simulink model "full_sim"  (R2020b)
settings: Solver=FixedStepAuto  StartTime=0.0  StopTime=inf  FixedStep=0.005  RelTol=1e-3
InitFcn:
  | % Load config data automatically
  | load("config.mat");
  | 
  | track = gen_track;
  | map = double(rgb2gray(imread('map.png')));%'iSpaceMapV2.0_50dpi.png')))*100/255;
StartFcn:
  | % The event listener triggers when the signal updates, so we can just monitor one of the signals.
  | blk1 = 'full_sim/GUI_update';
  | 
  | event = 'PostOutputs';
  | listener = @updateApp;
  | 
  | % Create the listener
  | h1 = add_exec_event_listener(blk1, event, listener);
StopFcn:
  | fclose('all') % close any log files that may still be open
model workspace (MAT data in the model file):
  ResetMode = "Reset at each sample time"
  initX = -0.39
  initY = 0.33
  initYaw = 3.14159265359
libraries: simulink x7, simulink_extras x6, dspnetwork x6, pid_lib x2, sldrtlib x1
CloseFcn:
  | fclose('all') % close any log files that may still be open
settings Model: Creator=Duncan  LastModifiedBy=dffleiss
settings DataIOCC: SaveOutput=off  SignalLogging=off  DSMLogging=off  SaveTime=off  ReturnWorkspaceOutputs=off
settings RTWCC: BuildConfiguration=Faster Runs

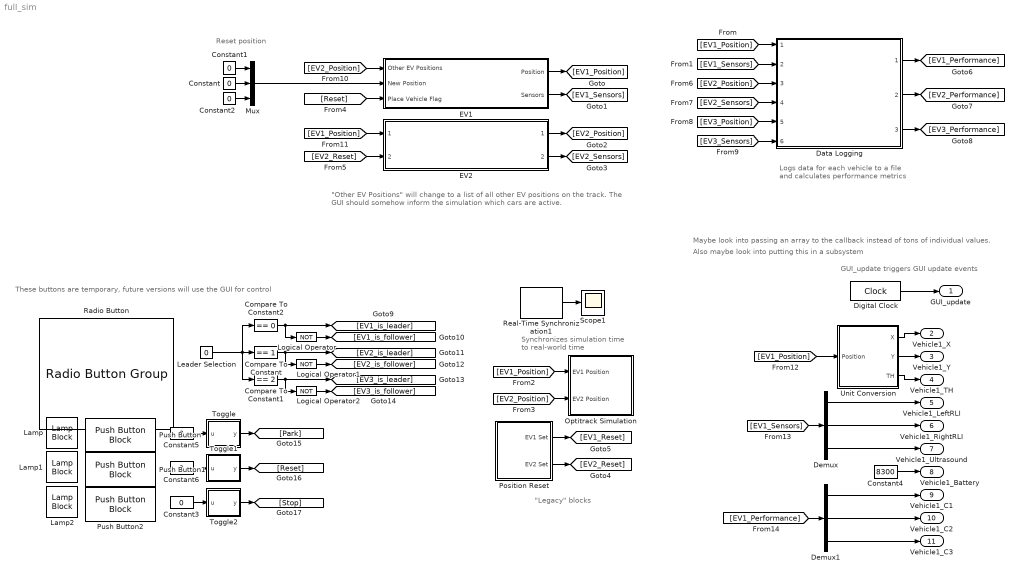
== system full_sim ==
  note: Reset position
  note: These buttons are temporary, future versions will use the GUI for control
  note: "Other EV Positions" will change to a list of all other EV positions on the track.
      | The GUI should somehow inform the simulation which cars are active.
  note: "Legacy" blocks
  note: Synchronizes simulation
      | time to real-world time
  note: Logs data for each vehicle to a file
      | and calculates performance metrics
  note: GUI_update triggers GUI update events
  note: Also maybe look into putting this in a subsystem
  note: Maybe look into passing an array to the callback instead of tons of individual values.
  Compare To Constant : simulink/Logic and Bit Operations/Compare To Constant  relop===  const=1  OutDataTypeStr=boolean
  Compare To Constant1 : simulink/Logic and Bit Operations/Compare To Constant  relop===  const=2  OutDataTypeStr=boolean
  Compare To Constant2 : simulink/Logic and Bit Operations/Compare To Constant  relop===  const=0  OutDataTypeStr=boolean
  Constant{,1..3,5..6} (6 alike) : Constant  Value=0
  Constant4 : Constant  Value=8300
  Data Logging : Subsystem  ReferencedSubsystem=Data_Logging
  Demux : Demux  Outputs=3
  Demux1 : Demux  Outputs=3
  Digital Clock : DigitalClock  SampleTime=0.1
  EV1 : Subsystem
  EV2 : Subsystem  ReferencedSubsystem=Vehicle_Sim  dataTXPort=25004  dataRXPort=25005  cmdPort=25006  initX=0  initY=.33  initYaw=pi  joystickRXPort=25008
  Lamp : LampBlock
  Lamp1 : LampBlock
  Lamp2 : LampBlock
  Leader Selection : Constant  Value=0
  Logical Operator : Logic  Operator=NOT  AllPortsSameDT=off  OutDataTypeStr=boolean
  Logical Operator1 : Logic  Operator=NOT  AllPortsSameDT=off  OutDataTypeStr=boolean
  Logical Operator2 : Logic  Operator=NOT  AllPortsSameDT=off  OutDataTypeStr=boolean
  Mux : Mux  Inputs=3
  Optitrack Simulation : Subsystem
  Position Reset : Subsystem
  Push Button : PushButtonBlock  ButtonText=Park
  Push Button1 : PushButtonBlock  ButtonText=Reset
  Push Button2 : PushButtonBlock  ButtonText=Stop
  Radio Button : RadioButtonGroup  SelectedLabel=EV1 Leader  ButtonGroupName=Group
      settings: Values={{'EV1 Leader', 'EV2 Leader', 'EV3 Leader'}, [0 1 2]}
  Real-Time Synchronization1 : sldrtlib/Real-Time Synchronization  SampleTime=.01  MaxMissedTicks=inf  ShowMissedTicks=on  YieldWhenWaiting=off
  Scope1 : Scope
  Toggle : MATLAB Function  TreatAsAtomicUnit=on
  Toggle1 : MATLAB Function  TreatAsAtomicUnit=on
  Toggle2 : MATLAB Function  TreatAsAtomicUnit=on
  Unit Conversion : Subsystem
  GUI_update : Outport
  Vehicle1_X : Outport  Port=2
  Vehicle1_Y : Outport  Port=3
  Vehicle1_TH : Outport  Port=4
  Vehicle1_LeftRLI : Outport  Port=5
  Vehicle1_RightRLI : Outport  Port=6
  Vehicle1_Ultrasound : Outport  Port=7
  Vehicle1_Battery : Outport  Port=8
  Vehicle1_C1 : Outport  Port=9
  Vehicle1_C2 : Outport  Port=10
  Vehicle1_C3 : Outport  Port=11
  wires:
  [EV2_Position] -> EV1/1(Other EV Positions)
  [EV1_Position] -> EV2/1
  EV2/1 -> [EV2_Position]
  Mux/1 -> EV1/2(New Position)
  EV1/2(Sensors) -> [EV1_Sensors]
  EV1/1(Position) -> [EV1_Position]
  EV2/2 -> [EV2_Sensors]
  Position Reset/2(EV2 Set) -> [EV2_Reset]
  [EV1_Position] -> Optitrack Simulation/1(EV1 Position)
  Position Reset/1(EV1 Set) -> [EV1_Reset]
  [EV2_Position] -> Optitrack Simulation/2(EV2 Position)
  Data Logging/1 -> [EV1_Performance]
  Data Logging/3 -> [EV3_Performance]
  [EV1_Position] -> Data Logging/1
  [EV2_Sensors] -> Data Logging/4
  [EV2_Position] -> Data Logging/3
  [EV3_Position] -> Data Logging/5
  Data Logging/2 -> [EV2_Performance]
  [EV3_Sensors] -> Data Logging/6
  [EV1_Sensors] -> Data Logging/2
  Real-Time Synchronization1/1 -> Scope1/1
  [EV1_Performance] -> Demux1/1
  Demux1/3 -> Vehicle1_C3/1
  Unit Conversion/1(X) -> Vehicle1_X/1
  Demux/2 -> Vehicle1_RightRLI/1
  Unit Conversion/2(Y) -> Vehicle1_Y/1
  Unit Conversion/3(TH) -> Vehicle1_TH/1
  Constant4/1 -> Vehicle1_Battery/1
  Demux1/1 -> Vehicle1_C1/1
  Demux/1 -> Vehicle1_LeftRLI/1
  [EV1_Position] -> Unit Conversion/1(Position)
  Digital Clock/1 -> GUI_update/1
  Demux1/2 -> Vehicle1_C2/1
  [EV1_Sensors] -> Demux/1
  Demux/3 -> Vehicle1_Ultrasound/1
  Constant2/1 -> Mux/3
  Constant/1 -> Mux/2
  Constant1/1 -> Mux/1
  Logical Operator1/1 -> [EV2_is_follower]
  Logical Operator/1 -> [EV1_is_follower]
  Compare To Constant2/1 -> [EV1_is_leader], Logical Operator/1
  Compare To Constant/1 -> [EV2_is_leader], Logical Operator1/1
  Logical Operator2/1 -> [EV3_is_follower]
  Compare To Constant1/1 -> [EV3_is_leader], Logical Operator2/1
  Leader Selection/1 -> Compare To Constant1/1, Compare To Constant2/1, Compare To Constant/1
  Toggle/1(y) -> [Park]
  Constant5/1 -> Toggle/1(u)
  Toggle1/1(y) -> [Reset]
  Constant6/1 -> Toggle1/1(u)
  Toggle2/1(y) -> [Stop]
  Constant3/1 -> Toggle2/1(u)
  [EV2_Reset] -> EV2/2
  [Reset] -> EV1/3(Place Vehicle Flag)

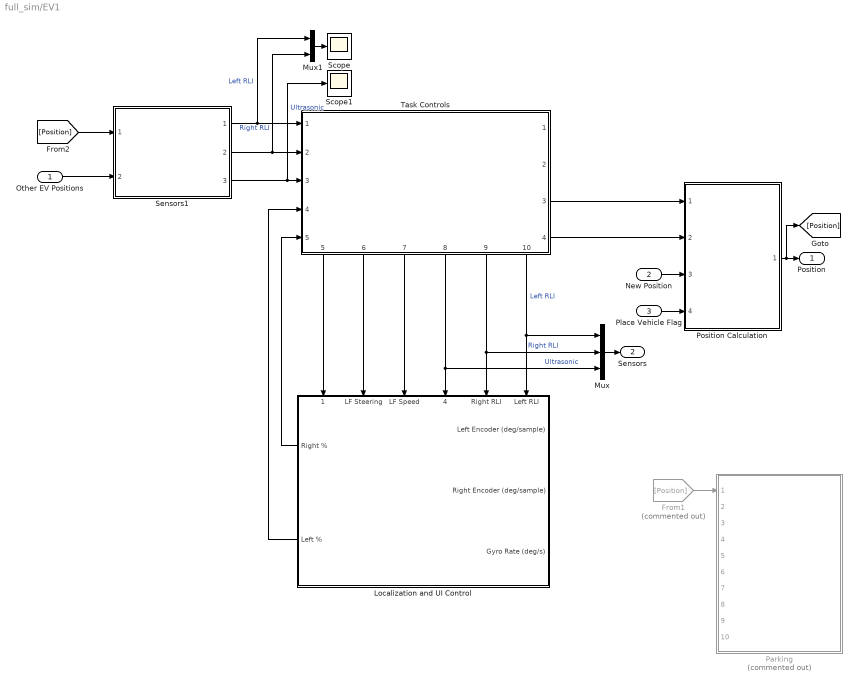
== system full_sim/EV1 ==
  Other EV Positions : Inport
  New Position : Inport  Port=2
  Place Vehicle Flag : Inport  Port=3
  From1 : From  Commented=on  GotoTag=Position
  Localization and UI Control : Subsystem
      settings: PortSchema="{\"entries\":[{\"content\":{\"sides\":[{\"content\":{\"connectorIds\":[\"Out1\",\"Out2\"]},\"type\":\"ConnectorPlacement.EquallySpacedRectSide\",\"uuid\":\"c41f9887-e70f-42cb-a70d-ce479c94e8e6\"},{\"content\":{\"connectorIds\":[\"In7\",\"In8\",\"In9\"],\"side\":\"RIGHT\"},\"type\":\"ConnectorPlacement.EquallySpacedRectSide\",\"uuid\":\"01fea69d-4e07-40c9-8b78-412f64609b36\"},{\"content\":{\"connectorIds\":[\"In1\",\"In2\",\"In3\",\"In4\",\"In5\",\"In6\"],\"side\":\"TOP\"},\"type\":\"ConnectorPlacement.EquallySpacedRectSide\",\"uuid\":\"d2fc7682-afac-46c9-9372-ea085883672c\"}]},\"type\":\"ConnectorPlacement.EquallySpacedConnector\",\"uuid\":\"f49fd9b7-3a1c-45a5-ac31-ef3904fd2313\"}],\"packageUris\":[\"http://schema.mathworks.com/mf0/Connector/19700101\"],\"version\":\"1.0\"}"
  Mux : Mux  Inputs=3
  Mux1 : Mux  Inputs=2
  Parking : Subsystem  Commented=on  ReferencedSubsystem=Parking_ThorneFleissner
  Position Calculation : Subsystem  ReferencedSubsystem=Position_Calculation_ThorneFleissner
  Scope : Scope
  Scope1 : Scope
  Sensors1 : Subsystem  ReferencedSubsystem=Sensors_ThorneFleissner
  Task Controls : Subsystem  ReferencedSubsystem=Task_Controls_ThorneFleissner
      settings: PortSchema="{\"entries\":[{\"content\":{\"sides\":[{\"content\":{\"connectorIds\":[\"In1\",\"In2\",\"In3\",\"In4\",\"In5\"]},\"type\":\"ConnectorPlacement.EquallySpacedRectSide\",\"uuid\":\"3c64813c-625d-49d1-ae67-306451c3c1fa\"},{\"content\":{\"connectorIds\":[\"Out1\",\"Out2\",\"Out3\",\"Out4\"],\"side\":\"RIGHT\"},\"type\":\"ConnectorPlacement.EquallySpacedRectSide\",\"uuid\":\"91793cf5-b7a0-4d71-a2c0-83cdd43afca2\"},{\"content\":{\"connectorIds\":[],\"side\":\"TOP\"},\"type\":\"ConnectorPlacement.EquallySpacedRectSide\",\"uuid\":\"5300aefe-28d7-4142-9759-b53f625cf082\"},{\"content\":{\"connectorIds\":[\"Out5\",\"Out6\",\"Out7\",\"Out8\",\"Out9\",\"Out10\"],\"side\":\"BOTTOM\"},\"type\":\"ConnectorPlacement.EquallySpacedRectSide\",\"uuid\":\"7541b0a2-c079-4b1b-9276-8e4ee5949dfd\"},{\"content\":{\"connectorIds\":[],\"side\":\"HIDDEN\"},\"type\":\"ConnectorPlacement.EquallySpacedRectSide\",\"uuid\":\"d0ef4c96-52b1-4a81-ac1e-c57b650a37a1\"}]},\"type\":\"ConnectorPlacement.EquallySpacedConnector\",\"uuid\":\"d02aae7f-e4d5-4935-81ce-eef5c5855771\"}],\"packageUris\":[\"http://schema.mathworks.com/mf0/Connector/R2020b\"],\"version\":\"1.0\"}"
  Position : Outport
  Sensors : Outport  Port=2
  wires:
  Localization and UI Control/2(Left %) -> Task Controls/4
  Other EV Positions/1 -> Sensors1/2
  Localization and UI Control/1(Right %) -> Task Controls/5
  Task Controls/4 -> Position Calculation/2
  Task Controls/3 -> Position Calculation/1
  Task Controls/7 -> Localization and UI Control/3(LF Speed)
  Task Controls/6 -> Localization and UI Control/2(LF Steering)
  Task Controls/5 -> Localization and UI Control/1(Platoon Speed)
  Task Controls/10 -> Localization and UI Control/6(Left RLI), Mux/1  "Left RLI"
  Task Controls/9 -> Localization and UI Control/5(Right RLI), Mux/2  "Right RLI"
  Task Controls/8 -> Localization and UI Control/4(Ultrasonic (cm)), Mux/3  "Ultrasonic"
  Sensors1/1 -> Mux1/1, Task Controls/1  "Left RLI"
  Sensors1/2 -> Mux1/2, Task Controls/2  "Right RLI"
  Sensors1/3 -> Scope1/1, Task Controls/3  "Ultrasonic"
  Mux/1 -> Sensors/1
  Place Vehicle Flag/1 -> Position Calculation/4
  New Position/1 -> Position Calculation/3
  From1/1 -> Parking/1
  [Position] -> Sensors1/1
  Position Calculation/1 -> [Position], Position/1
  Mux1/1 -> Scope/1

== system full_sim/Optitrack Simulation ==
  EV1 Position : Inport
  EV2 Position : Inport  Port=2
  MATLAB Function : MATLAB Function  TreatAsAtomicUnit=on
  UDP Send : dspnetwork/UDP Send  remoteURL='127.0.0.1'  remotePort=1511  localURL='0.0.0.0'  localPortSource=Automatically determine  localPort=-1  sendBufferSize=8192  sampletime=-1  blockPlatform=[]  separateLengthPort=0
  wires:
  EV1 Position/1 -> MATLAB Function/1(ev1pos)
  EV2 Position/1 -> MATLAB Function/2(ev2pos)
  MATLAB Function/1(packet) -> UDP Send/1

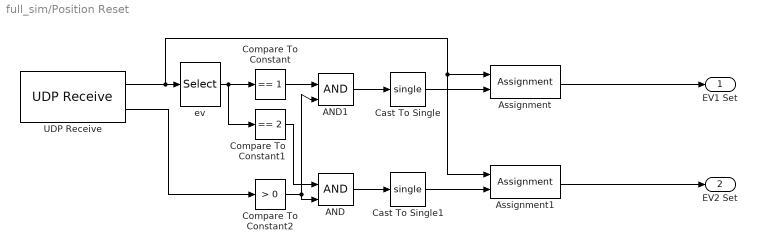
== system full_sim/Position Reset ==
  AND : Logic  IconShape=distinctive  AllPortsSameDT=off  OutDataTypeStr=boolean
  AND1 : Logic  IconShape=distinctive  AllPortsSameDT=off  OutDataTypeStr=boolean
  Assignment : Assignment  DiagnosticForDimensions=Warning  IndexOptions=Index vector (dialog)  Indices=1  OutputSizes=1
  Assignment1 : Assignment  DiagnosticForDimensions=Warning  IndexOptions=Index vector (dialog)  Indices=1  OutputSizes=1
  Cast To Single : DataTypeConversion  OutDataTypeStr=single
  Cast To Single1 : DataTypeConversion  OutDataTypeStr=single
  Compare To Constant : simulink/Logic and Bit Operations/Compare To Constant  relop===  const=1  OutDataTypeStr=boolean
  Compare To Constant1 : simulink/Logic and Bit Operations/Compare To Constant  relop===  const=2  OutDataTypeStr=boolean
  Compare To Constant2 : simulink/Logic and Bit Operations/Compare To Constant  relop=>  const=0  OutDataTypeStr=boolean
  UDP Receive : dspnetwork/UDP Receive  localURL='0.0.0.0'  localPort=24999  remoteURL='0.0.0.0'  remotePort=-1  recvBufferSize=512  dims=4  signalDatatype=single  isComplex=off  isVarSize=off  showBlockingTime=off  blockingTime=0  sampletime=0.01  blockPlatform=[]
  ev : Selector  InputPortWidth=4  IndexOptions=Index vector (dialog)  Indices=[1]  OutputSizes=1
  EV1 Set : Outport
  EV2 Set : Outport  Port=2
  wires:
  Compare To Constant2/1 -> AND1/2, AND/2
  UDP Receive/2 -> Compare To Constant2/1
  ev/1 -> Compare To Constant1/1, Compare To Constant/1
  Assignment/1 -> EV1 Set/1
  Compare To Constant/1 -> AND1/1
  Assignment1/1 -> EV2 Set/1
  UDP Receive/1 -> Assignment/1, Assignment1/1, ev/1
  AND/1 -> Cast To Single1/1
  Compare To Constant1/1 -> AND/1
  Cast To Single/1 -> Assignment/2
  AND1/1 -> Cast To Single/1
  Cast To Single1/1 -> Assignment1/2

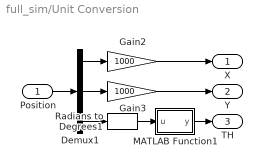
== system full_sim/Unit Conversion ==
  Position : Inport
  Demux1 : Demux  Outputs=3
  Gain2 : Gain  Gain=1000
  Gain3 : Gain  Gain=1000
  MATLAB Function1 : MATLAB Function  TreatAsAtomicUnit=on
  Radians to Degrees1 : simulink_extras/Transformations/Radians to Degrees
  X : Outport
  Y : Outport  Port=2
  TH : Outport  Port=3
  wires:
  Radians to Degrees1/1 -> MATLAB Function1/1(u)
  Gain3/1 -> Y/1
  Demux1/3 -> Radians to Degrees1/1
  Demux1/2 -> Gain3/1
  Gain2/1 -> X/1
  MATLAB Function1/1(y) -> TH/1
  Demux1/1 -> Gain2/1
  Position/1 -> Demux1/1

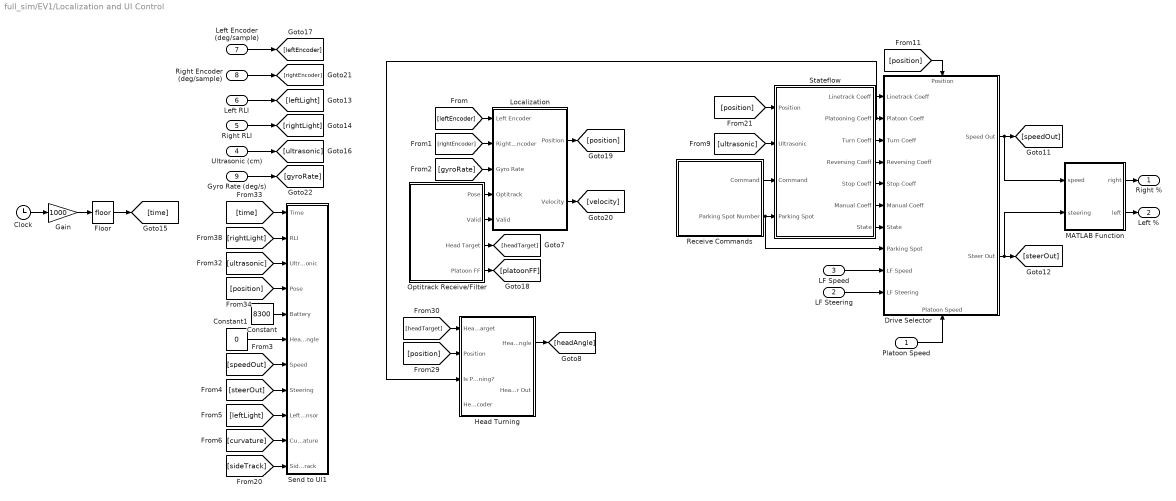
== system full_sim/EV1/Localization and UI Control ==
  Platoon Speed : Inport
  LF Steering : Inport  Port=2
  LF Speed : Inport  Port=3
  Ultrasonic (cm) : Inport  Port=4
  Right RLI : Inport  Port=5
  Left RLI : Inport  Port=6
  Left Encoder (deg/sample) : Inport  Port=7
  Right Encoder (deg/sample) : Inport  Port=8
  Gyro Rate (deg/s) : Inport  Port=9
  Clock : Clock
  Constant : Constant  Value=8300
  Constant1 : Constant  Value=0
  Drive Selector : Subsystem
      settings: PortSchema="{\"entries\":[{\"content\":{\"sides\":[{\"content\":{\"connectorIds\":[\"In1\",\"In2\",\"In3\",\"In4\",\"In5\",\"In6\",\"In7\",\"In8\",\"In9\",\"In10\"]},\"type\":\"ConnectorPlacement.EquallySpacedRectSide\",\"uuid\":\"ae307232-287c-4602-bc59-e7aee20cf720\"},{\"content\":{\"connectorIds\":[\"Out1\",\"Out2\"],\"side\":\"RIGHT\"},\"type\":\"ConnectorPlacement.EquallySpacedRectSide\",\"uuid\":\"2cae2544-d808-4029-9530-a1f56251b9cd\"},{\"content\":{\"connectorIds\":[\"In11\"],\"side\":\"TOP\"},\"type\":\"ConnectorPlacement.EquallySpacedRectSide\",\"uuid\":\"bbc0be7b-0147-487e-824e-99eef1e06dcc\"},{\"content\":{\"connectorIds\":[\"In12\"],\"side\":\"BOTTOM\"},\"type\":\"ConnectorPlacement.EquallySpacedRectSide\",\"uuid\":\"b1fbed80-afe2-48db-af11-c85938407aae\"}]},\"type\":\"ConnectorPlacement.EquallySpacedConnector\",\"uuid\":\"38f7d747-6147-4f1b-8575-02c2e0fe0660\"}],\"packageUris\":[\"http://schema.mathworks.com/mf0/Connector/19700101\"],\"version\":\"1.0\"}"
  Floor : Rounding
  Gain : Gain  Gain=1000
  Head Turning : Subsystem
  Localization : Subsystem
  MATLAB Function : MATLAB Function  TreatAsAtomicUnit=on
  Optitrack Receive/Filter : Subsystem
  Receive Commands : Subsystem
  Send to UI1 : Subsystem
  Stateflow : Subsystem
  Right % : Outport
  Left % : Outport  Port=2
  wires:
  Constant/1 -> Send to UI1/5(Battery)
  [position] -> Head Turning/2(Position)
  Left RLI/1 -> [leftLight]
  Localization/2(Velocity) -> [velocity]
  Stateflow/6(Manual Coeff) -> Drive Selector/6(Manual Coeff)
  [leftEncoder] -> Localization/1(Left Encoder)
  MATLAB Function/1(right) -> Right %/1
  Head Turning/1(Head Angle) -> [headAngle]
  Optitrack Receive/Filter/4(Platoon FF) -> [platoonFF]
  [gyroRate] -> Localization/3(Gyro Rate)
  Floor/1 -> [time]
  Drive Selector/2(Steer Out) -> [steerOut], MATLAB Function/2(steering)
  Optitrack Receive/Filter/2(Valid) -> Localization/5(Valid)
  Clock/1 -> Gain/1
  Right Encoder (deg/sample)/1 -> [rightEncoder]
  Optitrack Receive/Filter/3(Head Target) -> [headTarget]
  Left Encoder (deg/sample)/1 -> [leftEncoder]
  Gain/1 -> Floor/1
  Receive Commands/1(Command) -> Stateflow/3(Command)
  [ultrasonic] -> Send to UI1/3(Ultrasonic)
  [curvature] -> Send to UI1/10(Curvature)
  Stateflow/4(Reversing Coeff) -> Drive Selector/4(Reversing Coeff)
  Gyro Rate (deg/s)/1 -> [gyroRate]
  [leftLight] -> Send to UI1/9(Left Sensor)
  [sideTrack] -> Send to UI1/11(Side Track)
  Drive Selector/1(Speed Out) -> [speedOut], MATLAB Function/1(speed)
  Right RLI/1 -> [rightLight]
  Ultrasonic (cm)/1 -> [ultrasonic]
  MATLAB Function/2(left) -> Left %/1
  [speedOut] -> Send to UI1/7(Speed)
  [steerOut] -> Send to UI1/8(Steering)
  Stateflow/7(State) -> Drive Selector/7(State)
  Stateflow/5(Stop Coeff) -> Drive Selector/5(Stop Coeff)
  Localization/1(Position) -> [position]
  Optitrack Receive/Filter/1(Pose) -> Localization/4(Optitrack)
  [position] -> Send to UI1/4(Pose)
  Stateflow/3(Turn Coeff) -> Drive Selector/3(Turn Coeff)
  [rightLight] -> Send to UI1/2(RLI)
  Stateflow/2(Platooning Coeff) -> Head Turning/3(Is Platooning?), Drive Selector/2(Platoon Coeff)
  [ultrasonic] -> Stateflow/2(Ultrasonic)
  [headTarget] -> Head Turning/1(Head Target)
  [position] -> Stateflow/1(Position)
  Stateflow/1(Linetrack Coeff) -> Drive Selector/1(Linetrack Coeff)
  Receive Commands/2(Parking Spot Number) -> Drive Selector/8(Parking Spot), Stateflow/4(Parking Spot)
  [position] -> Drive Selector/11(Position)
  [rightEncoder] -> Localization/2(Right Encoder)
  [time] -> Send to UI1/1(Time)
  Constant1/1 -> Send to UI1/6(Head Angle)
  LF Speed/1 -> Drive Selector/9(LF Speed)
  LF Steering/1 -> Drive Selector/10(LF Steering)
  Platoon Speed/1 -> Drive Selector/12(Platoon Speed)

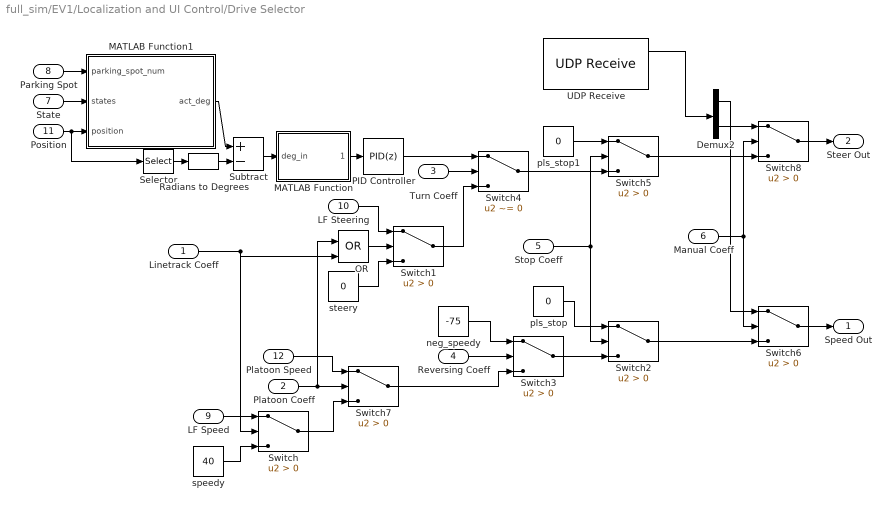
== system full_sim/EV1/Localization and UI Control/Drive Selector ==
  Linetrack Coeff : Inport
  Platoon Coeff : Inport  Port=2
  Turn Coeff : Inport  Port=3
  Reversing Coeff : Inport  Port=4
  Stop Coeff : Inport  Port=5
  Manual Coeff : Inport  Port=6
  State : Inport  Port=7
  Parking Spot : Inport  Port=8
  LF Speed : Inport  Port=9
  LF Steering : Inport  Port=10
  Position : Inport  Port=11
  Platoon Speed : Inport  Port=12
  Demux2 : Demux  Outputs=2
  MATLAB Function : MATLAB Function  TreatAsAtomicUnit=on
  MATLAB Function1 : MATLAB Function  TreatAsAtomicUnit=on
  OR : Logic  Operator=OR  IconShape=distinctive  AllPortsSameDT=off  OutDataTypeStr=boolean
  PID Controller : pid_lib/PID Controller  Controller=PID  Form=Parallel  TimeDomain=Discrete-time  UseExternalTs=off  SampleTime=-1  IntegratorMethod=Forward Euler  FilterMethod=Forward Euler  ControllerParametersSource=internal  P=1  I=0  D=0  UseFilter=off  N=100  TunerSelectOption=Transfer Function Based (PID Tuner App)  InitialConditionSource=internal  InitialConditionForIntegrator=0  InitialConditionForFilter=0  DifferentiatorICPrevScaledInput=0  ExternalReset=none  TrackingMode=off  Kt=1  LimitOutput=off  SatLimitsSource=internal  UpperSaturationLimit=inf  LowerSaturationLimit=-inf  LinearizeAsGain=on  AntiWindupMode=none  Kb=1  POutMin=[]  POutMax=[]  IOutMin=[]  IOutMax=[]  DOutMin=[]  DOutMax=[]  NOutMin=[]  NOutMax=[]  SumOutMin=[]  SumOutMax=[]  SaturationOutMin=[]  SaturationOutMax=[]  PParamMin=[]  PParamMax=[]  IParamMin=[]  IParamMax=[]  DParamMin=[]  DParamMax=[]  NParamMin=[]  NParamMax=[]  KbParamMin=[]  KbParamMax=[]  KtParamMin=[]  KtParamMax=[]  KbOutMin=[]  KbOutMax=[]  KtOutMin=[]  KtOutMax=[]  IntegratorOutMin=[]  IntegratorOutMax=[]  FilterOutMin=[]  FilterOutMax=[]  SumI1OutMin=[]  SumI1OutMax=[]  SumI2OutMin=[]  SumI2OutMax=[]  SumI3OutMin=[]  SumI3OutMax=[]  SumI4OutMin=[]  SumI4OutMax=[]  SumDOutMin=[]  SumDOutMax=[]  DifferentiatorOutMin=[]  DifferentiatorOutMax=[]  FilterDiffOutCoefMin=[]  FilterDiffOutCoefMax=[]  ReciprocalOutMin=[]  ReciprocalOutMax=[]  SumDenOutMin=[]  SumDenOutMax=[]  SumNumOutMin=[]  SumNumOutMax=[]  DivideOutMin=[]  DivideOutMax=[]  UdiffTsProdOutMin=[]  UdiffTsProdOutMax=[]  NTsProdOutMin=[]  NTsProdOutMax=[]  UintegralTsProdOutMin=[]  UintegralTsProdOutMax=[]  UngainTsProdOutMin=[]  UngainTsProdOutMax=[]  IntegratorContinuousStateAttributes=''  IntegratorStateMustResolveToSignalObject=off  IntegratorRTWStateStorageClass=Auto  FilterContinuousStateAttributes=''  FilterStateMustResolveToSignalObject=off  FilterRTWStateStorageClass=Auto  ParallelPVariant=InternalParameters  IdealPVariant=Disabled  IVariant=InternalParameters  DVariant=InternalParameters  IntegratorVariant=Discrete  SatVariant=Disabled  AWVariant=Passthrough  PCopyVariant=Disabled  TRVariant=Disabled  FdbkBlocksVariant=Forward  IdealPFdbkVariant=Disabled  SatFdbkVariant=Disabled  DerivativeFilterVariant=Differentiator  NVariant=Passthrough  NCopyVariant=Disabled_SignalSpec  FilterICVariant=InternalICsDifferentiator  IntegratorICVariant=InternalICs  ExternalResetVariant=Disabled  TRSumVariant=Passthrough  SumFdbkVariant=Disabled  SumVariant=Sum_PID  TsampFilterVariant=InternalTs  TsampNgainVariant=Passthrough  TsampIntegralVariant=Passthrough  ExternalSaturationOutDataTypeStr=Inherit: Same as second input
  Radians to Degrees : simulink_extras/Transformations/Radians to Degrees
  Selector : Selector  InputPortWidth=3  IndexOptions=Index vector (dialog)  Indices=[3]  OutputSizes=1
  Subtract : Sum  Inputs=+-
  Switch{,1..3,5..8} (8 alike) : Switch  Criteria=u2 > Threshold
  Switch4 : Switch  Criteria=u2 ~= 0
  UDP Receive : dspnetwork/UDP Receive  localURL='0.0.0.0'  localPort=joystickRXPort  remoteURL='0.0.0.0'  remotePort=-1  recvBufferSize=384  dims=2  signalDatatype=single  isComplex=off  isVarSize=off  showBlockingTime=off  blockingTime=0  sampletime=0.01  blockPlatform=[]
  neg_speedy : Constant  Value=-75
  pls_stop : Constant  Value=0
  pls_stop1 : Constant  Value=0
  speedy : Constant  Value=40
  steery : Constant  Value=0
  Speed Out : Outport
  Steer Out : Outport  Port=2
  wires:
  Demux2/1 -> Switch6/1
  Demux2/2 -> Switch8/1
  Switch6/1 -> Speed Out/1
  Switch8/1 -> Steer Out/1
  Manual Coeff/1 -> Switch6/2, Switch8/2
  Switch2/1 -> Switch6/3
  Switch5/1 -> Switch8/3
  UDP Receive/1 -> Demux2/1
  LF Speed/1 -> Switch/1
  LF Steering/1 -> Switch1/1
  steery/1 -> Switch1/3
  speedy/1 -> Switch/3
  Switch1/1 -> Switch4/3
  Switch3/1 -> Switch2/3
  Stop Coeff/1 -> Switch2/2, Switch5/2
  pls_stop/1 -> Switch2/1
  Turn Coeff/1 -> Switch4/2
  PID Controller/1 -> Switch4/1
  Subtract/1 -> MATLAB Function/1(deg_in)
  MATLAB Function/1(deg_out) -> PID Controller/1
  Radians to Degrees/1 -> Subtract/2
  Parking Spot/1 -> MATLAB Function1/1(parking_spot_num)
  Reversing Coeff/1 -> Switch3/2
  State/1 -> MATLAB Function1/2(states)
  Position/1 -> Selector/1, MATLAB Function1/3(position)
  Switch4/1 -> Switch5/3
  neg_speedy/1 -> Switch3/1
  MATLAB Function1/1(act_deg) -> Subtract/1
  OR/1 -> Switch1/2
  Platoon Coeff/1 -> OR/1, Switch7/2
  Linetrack Coeff/1 -> Switch/2, OR/2
  Switch7/1 -> Switch3/3
  Switch/1 -> Switch7/3
  Selector/1 -> Radians to Degrees/1
  pls_stop1/1 -> Switch5/1
  Platoon Speed/1 -> Switch7/1

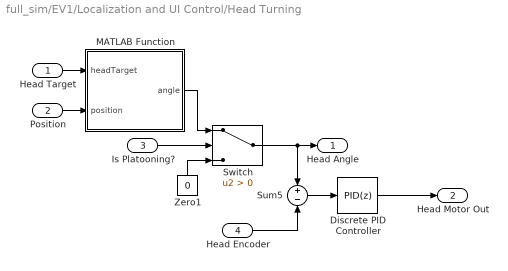
== system full_sim/EV1/Localization and UI Control/Head Turning ==
  Head Target : Inport
  Position : Inport  Port=2
  Is Platooning? : Inport  Port=3
  Head Encoder : Inport  Port=4
  Discrete PID Controller : pid_lib/PID Controller  Controller=PID  Form=Parallel  TimeDomain=Discrete-time  UseExternalTs=off  SampleTime=-1  IntegratorMethod=Forward Euler  FilterMethod=Forward Euler  ControllerParametersSource=internal  P=1  I=1  D=0  UseFilter=off  N=100  TunerSelectOption=Transfer Function Based (PID Tuner App)  InitialConditionSource=internal  InitialConditionForIntegrator=0  InitialConditionForFilter=0  DifferentiatorICPrevScaledInput=0  ExternalReset=none  TrackingMode=off  Kt=1  LimitOutput=off  SatLimitsSource=internal  UpperSaturationLimit=inf  LowerSaturationLimit=-inf  LinearizeAsGain=off  AntiWindupMode=none  Kb=1  POutMin=[]  POutMax=[]  IOutMin=[]  IOutMax=[]  DOutMin=[]  DOutMax=[]  NOutMin=[]  NOutMax=[]  SumOutMin=[]  SumOutMax=[]  SaturationOutMin=[]  SaturationOutMax=[]  PParamMin=[]  PParamMax=[]  IParamMin=[]  IParamMax=[]  DParamMin=[]  DParamMax=[]  NParamMin=[]  NParamMax=[]  KbParamMin=[]  KbParamMax=[]  KtParamMin=[]  KtParamMax=[]  KbOutMin=[]  KbOutMax=[]  KtOutMin=[]  KtOutMax=[]  IntegratorOutMin=[]  IntegratorOutMax=[]  FilterOutMin=[]  FilterOutMax=[]  SumI1OutMin=[]  SumI1OutMax=[]  SumI2OutMin=[]  SumI2OutMax=[]  SumI3OutMin=[]  SumI3OutMax=[]  SumI4OutMin=[]  SumI4OutMax=[]  SumDOutMin=[]  SumDOutMax=[]  DifferentiatorOutMin=[]  DifferentiatorOutMax=[]  FilterDiffOutCoefMin=[]  FilterDiffOutCoefMax=[]  ReciprocalOutMin=[]  ReciprocalOutMax=[]  SumDenOutMin=[]  SumDenOutMax=[]  SumNumOutMin=[]  SumNumOutMax=[]  DivideOutMin=[]  DivideOutMax=[]  UdiffTsProdOutMin=[]  UdiffTsProdOutMax=[]  NTsProdOutMin=[]  NTsProdOutMax=[]  UintegralTsProdOutMin=[]  UintegralTsProdOutMax=[]  UngainTsProdOutMin=[]  UngainTsProdOutMax=[]  IntegratorContinuousStateAttributes=''  IntegratorStateMustResolveToSignalObject=off  IntegratorRTWStateStorageClass=Auto  FilterContinuousStateAttributes=''  FilterStateMustResolveToSignalObject=off  FilterRTWStateStorageClass=Auto  ParallelPVariant=InternalParameters  IdealPVariant=Disabled  IVariant=InternalParameters  DVariant=InternalParameters  IntegratorVariant=Discrete  SatVariant=Disabled  AWVariant=Passthrough  PCopyVariant=Disabled  TRVariant=Disabled  FdbkBlocksVariant=Forward  IdealPFdbkVariant=Disabled  SatFdbkVariant=Disabled  DerivativeFilterVariant=Differentiator  NVariant=Passthrough  NCopyVariant=Disabled_SignalSpec  FilterICVariant=InternalICsDifferentiator  IntegratorICVariant=InternalICs  ExternalResetVariant=Disabled  TRSumVariant=Passthrough  SumFdbkVariant=Disabled  SumVariant=Sum_PID  TsampFilterVariant=InternalTs  TsampNgainVariant=Passthrough  TsampIntegralVariant=Passthrough  ExternalSaturationOutDataTypeStr=Inherit: Same as second input
  MATLAB Function : MATLAB Function  TreatAsAtomicUnit=on
  Sum5 : Sum  Inputs=+|-
  Switch : Switch  Criteria=u2 > Threshold
  Zero1 : Constant  Value=0  OutDataTypeStr=Inherit: Inherit via back propagation
  Head Angle : Outport
  Head Motor Out : Outport  Port=2
  wires:
  Head Encoder/1 -> Sum5/2
  Position/1 -> MATLAB Function/2(position)
  Sum5/1 -> Discrete PID Controller/1
  Zero1/1 -> Switch/3
  Switch/1 -> Head Angle/1, Sum5/1
  Discrete PID Controller/1 -> Head Motor Out/1
  Head Target/1 -> MATLAB Function/1(headTarget)
  MATLAB Function/1(angle) -> Switch/1
  Is Platooning?/1 -> Switch/2

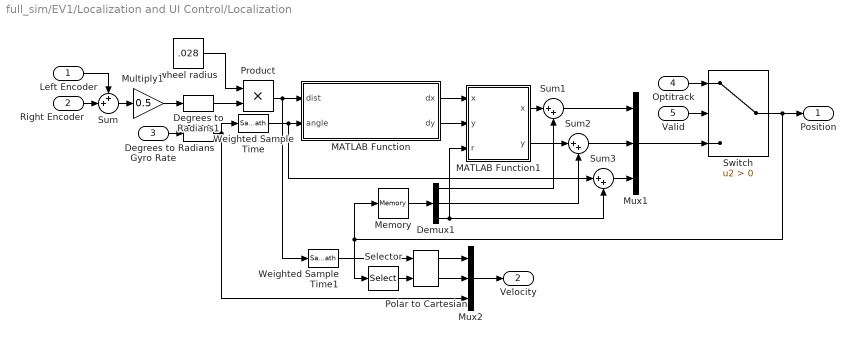
== system full_sim/EV1/Localization and UI Control/Localization ==
  Left Encoder : Inport
  Right Encoder : Inport  Port=2
  Gyro Rate : Inport  Port=3
  Optitrack : Inport  Port=4
  Valid : Inport  Port=5
  Degrees to Radians : simulink_extras/Transformations/Degrees to Radians
  Degrees to Radians1 : simulink_extras/Transformations/Degrees to Radians
  Demux1 : Demux  Outputs=3
  MATLAB Function : MATLAB Function  TreatAsAtomicUnit=on
  MATLAB Function1 : MATLAB Function  TreatAsAtomicUnit=on
  Memory : Memory
  Multiply1 : Gain  Gain=0.5
  Mux1 : Mux  Inputs=3
  Mux2 : Mux  Inputs=3
  Polar to Cartesian : simulink_extras/Transformations/Polar to Cartesian
      settings: SourceProductBaseCode=SL
  Product : Product
  Selector : Selector  InputPortWidth=3  IndexOptions=Index vector (dialog)  Indices=[3]  OutputSizes=1
  Sum : Sum  Inputs=++|
  Sum1 : Sum  Inputs=|++
  Sum2 : Sum  Inputs=|++
  Sum3 : Sum  Inputs=|++
  Switch : Switch  Criteria=u2 > Threshold
  Weighted Sample Time : SampleTimeMath  TsampMathOp=*
  Weighted Sample Time1 : SampleTimeMath  TsampMathOp=/
  wheel radius : Constant  Value=.028
  Position : Outport
  Velocity : Outport  Port=2
  wires:
  Sum/1 -> Multiply1/1
  MATLAB Function/1(dx) -> MATLAB Function1/1("x ")
  MATLAB Function/2(dy) -> MATLAB Function1/2("y ")
  Memory/1 -> Demux1/1
  Demux1/3 -> MATLAB Function1/3(r), Sum3/2
  MATLAB Function1/1(x) -> Sum1/1
  MATLAB Function1/2(y) -> Sum2/1
  Demux1/1 -> Sum1/2
  Demux1/2 -> Sum2/2
  Sum1/1 -> Mux1/1
  Sum2/1 -> Mux1/2
  Sum3/1 -> Mux1/3
  Left Encoder/1 -> Sum/1
  Right Encoder/1 -> Sum/2
  Gyro Rate/1 -> Degrees to Radians/1
  Degrees to Radians/1 -> Mux2/3, Weighted Sample Time/1
  Weighted Sample Time/1 -> Sum3/1, MATLAB Function/2(angle)
  Mux1/1 -> Switch/3
  Valid/1 -> Switch/2
  Optitrack/1 -> Switch/1
  Switch/1 -> Position/1, Memory/1, Selector/1
  Selector/1 -> Polar to Cartesian/2
  Polar to Cartesian/1 -> Mux2/1
  Polar to Cartesian/2 -> Mux2/2
  Mux2/1 -> Velocity/1
  Weighted Sample Time1/1 -> Polar to Cartesian/1
  Multiply1/1 -> Degrees to Radians1/1
  Product/1 -> Weighted Sample Time1/1, MATLAB Function/1(dist)
  Degrees to Radians1/1 -> Product/2
  wheel radius/1 -> Product/1

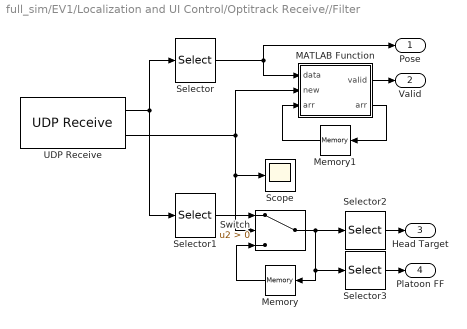
== system full_sim/EV1/Localization and UI Control/Optitrack Receive//Filter ==
  MATLAB Function : MATLAB Function  TreatAsAtomicUnit=on
  Memory : Memory
  Memory1 : Memory
  Scope : Scope
  Selector : Selector  InputPortWidth=6  IndexOptions=Index vector (dialog)  Indices=[1:3]  OutputSizes=1
  Selector1 : Selector  InputPortWidth=6  IndexOptions=Index vector (dialog)  Indices=[4:6]  OutputSizes=1
  Selector2 : Selector  InputPortWidth=3  IndexOptions=Index vector (dialog)  Indices=[1:2]  OutputSizes=1
  Selector3 : Selector  InputPortWidth=3  IndexOptions=Index vector (dialog)  Indices=[3]  OutputSizes=1
  Switch : Switch  Criteria=u2 > Threshold
  UDP Receive : dspnetwork/UDP Receive  localURL='0.0.0.0'  localPort=dataRXPort  remoteURL='0.0.0.0'  remotePort=-1  recvBufferSize=384  dims=6  signalDatatype=single  isComplex=off  isVarSize=off  showBlockingTime=off  blockingTime=0  sampletime=0.01  blockPlatform=[]
  Pose : Outport
  Valid : Outport  Port=2
  Head Target : Outport  Port=3
  Platoon FF : Outport  Port=4
  wires:
  MATLAB Function/1(valid) -> Valid/1
  MATLAB Function/2(arr) -> Memory1/1
  Memory1/1 -> MATLAB Function/3("arr ")
  Selector/1 -> Pose/1, MATLAB Function/1(data)
  Memory/1 -> Switch/3
  Switch/1 -> Selector2/1, Selector3/1, Memory/1
  Selector1/1 -> Switch/1
  UDP Receive/1 -> Selector/1, Selector1/1
  Selector2/1 -> Head Target/1
  Selector3/1 -> Platoon FF/1
  UDP Receive/2 -> Scope/1, Switch/2, MATLAB Function/2(new)

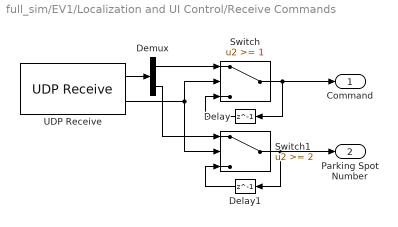
== system full_sim/EV1/Localization and UI Control/Receive Commands ==
  Delay : Delay  DelayLength=1  InitialCondition=0
  Delay1 : Delay  DelayLength=1  InitialCondition=0
  Demux : Demux  Outputs=2
  Switch : Switch  Threshold=1
  Switch1 : Switch  Threshold=2
  UDP Receive : dspnetwork/UDP Receive  localURL='0.0.0.0'  localPort=cmdPort  remoteURL='0.0.0.0'  remotePort=-1  recvBufferSize=384  dims=2  signalDatatype=uint8  isComplex=off  isVarSize=off  showBlockingTime=off  blockingTime=0  sampletime=0.01  blockPlatform=[]
  Command : Outport
  Parking Spot Number : Outport  Port=2
  wires:
  UDP Receive/2 -> Switch/2, Switch1/2
  UDP Receive/1 -> Demux/1
  Demux/1 -> Switch/1
  Switch/1 -> Command/1, Delay/1
  Delay/1 -> Switch/3
  Switch1/1 -> Parking Spot Number/1, Delay1/1
  Delay1/1 -> Switch1/3
  Demux/2 -> Switch1/1

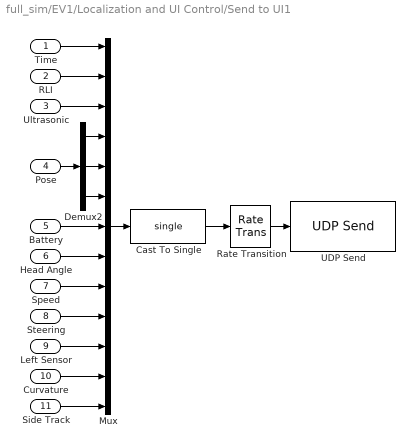
== system full_sim/EV1/Localization and UI Control/Send to UI1 ==
  Time : Inport
  RLI : Inport  Port=2
  Ultrasonic : Inport  Port=3
  Pose : Inport  Port=4
  Battery : Inport  Port=5
  Head Angle : Inport  Port=6
  Speed : Inport  Port=7
  Steering : Inport  Port=8
  Left Sensor : Inport  Port=9
  Curvature : Inport  Port=10
  Side Track : Inport  Port=11
  Cast To Single : DataTypeConversion  OutDataTypeStr=single
  Demux2 : Demux  Outputs=3
  Mux : Mux  Inputs=13
  Rate Transition : RateTransition  OutPortSampleTime=.04
  UDP Send : dspnetwork/UDP Send  remoteURL='127.0.0.1'  remotePort=dataTXPort  localURL='0.0.0.0'  localPortSource=Automatically determine  localPort=-1  sendBufferSize=8192  sampletime=-1  blockPlatform=[]  separateLengthPort=0
  wires:
  Rate Transition/1 -> UDP Send/1
  Demux2/1 -> Mux/4
  Ultrasonic/1 -> Mux/3
  Pose/1 -> Demux2/1
  Battery/1 -> Mux/7
  Mux/1 -> Cast To Single/1
  Demux2/2 -> Mux/5
  Demux2/3 -> Mux/6
  RLI/1 -> Mux/2
  Cast To Single/1 -> Rate Transition/1
  Time/1 -> Mux/1
  Speed/1 -> Mux/9
  Head Angle/1 -> Mux/8
  Steering/1 -> Mux/10
  Left Sensor/1 -> Mux/11
  Curvature/1 -> Mux/12
  Side Track/1 -> Mux/13

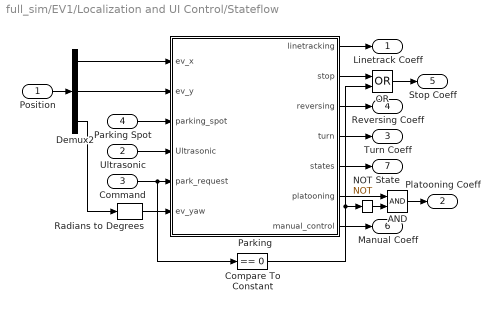
== system full_sim/EV1/Localization and UI Control/Stateflow ==
  Position : Inport
  Ultrasonic : Inport  Port=2
  Command : Inport  Port=3
  Parking Spot : Inport  Port=4
  AND : Logic  IconShape=distinctive  AllPortsSameDT=off  OutDataTypeStr=boolean
  Compare To Constant : simulink/Logic and Bit Operations/Compare To Constant  relop===  const=0  OutDataTypeStr=boolean
  Demux2 : Demux  Outputs=3
  NOT : Logic  Operator=NOT  IconShape=distinctive  AllPortsSameDT=off  OutDataTypeStr=boolean
  OR : Logic  Operator=OR  IconShape=distinctive  AllPortsSameDT=off  OutDataTypeStr=boolean
  Parking : Stateflow chart  TreatAsAtomicUnit=on
  Radians to Degrees : simulink_extras/Transformations/Radians to Degrees
  Linetrack Coeff : Outport
  Platooning Coeff : Outport  Port=2
  Turn Coeff : Outport  Port=3
  Reversing Coeff : Outport  Port=4
  Stop Coeff : Outport  Port=5
  Manual Coeff : Outport  Port=6
  State : Outport  Port=7
  wires:
  NOT/1 -> AND/2
  AND/1 -> Platooning Coeff/1
  Parking/6(platooning) -> AND/1
  Compare To Constant/1 -> OR/2, NOT/1
  Parking/2(stop) -> OR/1
  OR/1 -> Stop Coeff/1
  Parking/7(manual_control) -> Manual Coeff/1
  Demux2/3 -> Radians to Degrees/1
  Ultrasonic/1 -> Parking/4(Ultrasonic)
  Parking/1(linetracking) -> Linetrack Coeff/1
  Demux2/2 -> Parking/2(ev_y)
  Parking/3(reversing) -> Reversing Coeff/1
  Parking Spot/1 -> Parking/3(parking_spot)
  Demux2/1 -> Parking/1(ev_x)
  Parking/4(turn) -> Turn Coeff/1
  Position/1 -> Demux2/1
  Parking/5(states) -> State/1
  Radians to Degrees/1 -> Parking/6(ev_yaw)
  Command/1 -> Parking/5(park_request), Compare To Constant/1

== matlab function full_sim/Toggle ==
  data: u input; y output
function y = fcn(u)
    persistent state
    persistent button_pressed
    if isempty(state)
        state = false;
        button_pressed = false;
    end
    if u == 1 % u == 1 when button is pressed
        if ~button_pressed
            state = xor(state, 1); % toggle the output value
        end
        button_pressed = true; % prevent continuously toggling while button is pressed
    else
        button_pressed = false; % allow toggling after button has been released
    end
y = state;

== matlab function full_sim/Toggle1 ==
  data: u input; y output
function y = fcn(u)
    persistent state
    persistent button_pressed
    if isempty(state)
        state = false;
        button_pressed = false;
    end
    if u == 1 % u == 1 when button is pressed
        if ~button_pressed
            state = xor(state, 1); % toggle the output value
        end
        button_pressed = true; % prevent continuously toggling while button is pressed
    else
        button_pressed = false; % allow toggling after button has been released
    end
y = state;

== matlab function full_sim/Toggle2 ==
  data: u input; y output
function y = fcn(u)
    persistent state
    persistent button_pressed
    if isempty(state)
        state = false;
        button_pressed = false;
    end
    if u == 1 % u == 1 when button is pressed
        if ~button_pressed
            state = xor(state, 1); % toggle the output value
        end
        button_pressed = true; % prevent continuously toggling while button is pressed
    else
        button_pressed = false; % allow toggling after button has been released
    end
y = state;

== matlab function full_sim/Optitrack Simulation/MATLAB Function ==
  data: ev1pos input; packet output size=272; ev2pos input
function packet = fcn(ev1pos, ev2pos)
evs = {ev1pos,ev2pos};

packet = zeros(272,1,'uint8');

packet(1:2) = typecast(int16(7), 'uint8'); % packet type 
packet(17:20) = typecast(int32(length(evs)), 'uint8'); % num rigid bodies

for i = 1:length(evs)
    ptr = 21 + ((i-1)*120);
    pos = evs{i};
    q = eul2quat([pos(3),0,0]);
    % x, y, z, qx, qy, qz, qw
    packet(ptr+4:ptr+31) = typecast(single([pos(1) 0 pos(2) q(2) q(4) q(3) q(1)]), 'uint8');
end

== matlab function full_sim/Unit Conversion/MATLAB Function1 ==
  data: u input; y output
function y = fcn(u)
% Converts from infinite degrees to +/-180 degrees yaw
    new_angle = mod(u, 360);
    if new_angle > 180.0
        new_angle = new_angle - 360.0;
    end
    y = new_angle;
end

== matlab function full_sim/EV1/Localization and UI Control/Drive Selector/MATLAB Function ==
  data: deg_in input; deg_out output
function deg_out = remainder(deg_in)

deg_out = mod(deg_in+180,360)-180;

== matlab function full_sim/EV1/Localization and UI Control/Drive Selector/MATLAB Function1 ==
  data: parking_spot_num input; act_deg output; states input; position input
function act_deg = atan_me(parking_spot_num, states, position)

if parking_spot_num ==1 && states == 10
    degg = atan2(1.8-position(2), 0-position(1)); 
    
elseif parking_spot_num ==2 && states ==10
    degg = atan2(1.525 - position(2), 0-position(1));
    
elseif parking_spot_num ==3 && states == 10
    degg = atan2(1.1 - position(2), 0-position(1));
    
elseif parking_spot_num == 1 && states == 20
    %go to parking spot 1
    degg= atan2(1.6-position(2), -0.45-position(1)); 
%     degg = -168;
    
elseif parking_spot_num ==2 && states == 20
     %go to parking spot 2
    degg =atan2(1.2-position(2), -0.75-position(1)); 
%     degg = -165;
    
elseif parking_spot_num ==3 && states == 20 
    %go to parkin spot 3
    degg = atan2(0.80-position(2), -0.85-position(1)); 
%     degg = -150;
elseif parking_spot_num ~=0 && states == 30
    %complete parking and move angle to 180 degrees
    degg = pi; 
    
elseif parking_spot_num ~=0 && states == 40 
    %go to stop sign
    degg = atan2(0.525-position(2),0.0935-position(1)); 
    
elseif parking_spot_num ~=0 && states == 50
    degg = atan2(0.33 - position(2), -0.3 - position(1));
    %degg = -90; 
    
else
    degg = 0;
end 
act_deg = rad2deg(degg);
%act_deg = degg;

== matlab function full_sim/EV1/Localization and UI Control/Head Turning/MATLAB Function ==
  data: headTarget input; angle output; position input
function angle = headAngle(headTarget, position)

diff = headTarget - position(1:2);
angle = -double(rad2deg(atan2(diff(2),diff(1))-position(3)));
angle = mod(angle+180, 360) - 180;

== matlab function full_sim/EV1/Localization and UI Control/Localization/MATLAB Function ==
  data: dx output; dist input; angle input; dy output
function [dx,dy] = arc_approximation(dist,angle)
    if angle == 0
        dx = dist;
        dy = 0;
    else
        dx = sin(angle) * dist / angle;
        dy = (1-cos(angle)) * dist / angle;
    end

== matlab function full_sim/EV1/Localization and UI Control/Localization/MATLAB Function1 ==
  data: x input; x output; y input; r input; y output
function [x,y] = rotate2d(x,y,r)
    rot = [cos(r) -sin(r); sin(r) cos(r)] * [x;y];
    x = rot(1);
    y = rot(2);

== matlab function full_sim/EV1/Localization and UI Control/MATLAB Function ==
  data: right output; speed input; left output; steering input
function [right, left]= toMotorSpeeds(speed, steering)

left = speed - steering;
right = speed + steering;

m = max(left,right);
if m > 100
    left = left - m + 100;
    right = right - m + 100;
end

== matlab function full_sim/EV1/Localization and UI Control/Optitrack Receive//Filter/MATLAB Function ==
  data: data input; new input; arr input; valid output boolean; arr output
function [valid, arr]= filter(data,new,arr)

valid = false;
if new
    arr = circshift(arr,1);
    arr(1) = data(3);
    d = diff(arr);
    d = d - 2*pi*round(d/(2*pi));
    valid = all(abs(d) < deg2rad(5), 'all');
end

== stateflow chart full_sim/EV1/Localization and UI Control/Stateflow/Parking ==
  settings: executeAtInitialization=1
  state Leader_Goto_Intersection
    entry:
    linetracking =1;
    platooning =0;
    reversing = 0;
    turn = 0;
    stop =0;
    states = 10000;
  state Follower_Goto_Intersection
    entry:
    linetracking = 0;
    platooning =1;
    reversing = 0;
    turn =0;
    stop =0;
    states = 01000;
  state Enter_ParkingArea
    %Turn car 90 degrees
    entry:
    linetracking = 0;
    platooning =0;
    reversing = 0;
    turn = -1;
    stop =0;
    states = 00010;
  state Find_ParkingSpot
    entry:
    linetracking = 0;
    platooning  =0;
    reversing = 0;
    turn =2;
    stop = 0;
    states = 00020;
    %turn = 2 means find park (step 2 in turning)
    %Use the center of the target values to solve for the desired yaw that we want
    % Parking Spot 1 : x_cent = -0.45 ; y_cent =  1.6
    %Parking Spot 2: x_cent = -0.75; y_cent = 1.2
    %Parking Spot 3: x_cent = -0.85; y_cent = 0.80
  state Parking
    entry:
    linetracking = 0;
    platooning = 0;
    reversing = 0;
    turn=3;
    stop = 0;
    states = 00030;
    %turn =3 means 180 degrees
    %parking means to slow down the motor speed,
    %and to use ultrasonic sensor to detect for wall to stop
    %If ultrasonic sensor reaches a range of values-->parked
  state Parked
    entry:
    linetracking = 0;
    platooning = 0;
    reversing = 0;
    turn=0;
    stop = 1;
    states = 00001;
    %stop the car
  state Manual_Control
    entry:
    manual_control = 1;
    states = 100000;
    exit:
    manual_control = 0;
  state Reverse_Out_Spot
    entry:
    linetracking = 0;
    platooning = 0;
    reversing = 1;
    turn = 0;
    stop = 0;
    states = 00100;
    %once we find coordinate spot b we can
    %get rid of line tracking
  state Goto_Stop_Sign
    entry:
    linetracking = 0;
    platooning =0;
    reversing = 0;
    turn = 4;
    stop = 0;
    states = 00040;
    %turn = 4 means parking sign angle
  state Turn_Car_toInter
    %turn car -90 degrees
    entry:
    linetracking = 0;
    platooning =0;
    reversing = 0;
    turn = 5;
    stop = 0;
    states = 00050;
  state Finished
    entry:
    linetracking = 1;
    platooning =0;
    reversing = 0;
    turn =0;
    stop = 0;
    states = 10000;
    %can continue to linetrack the path.
  Manual_Control -> Leader_Goto_Intersection : [park_request ~= 4]
  Finished -> Leader_Goto_Intersection [order 1]
  (default) -> Leader_Goto_Intersection
  Leader_Goto_Intersection -> Follower_Goto_Intersection [order 1] : [park_request ==2]
  Leader_Goto_Intersection -> Manual_Control [order 3] : [park_request == 4]
  Follower_Goto_Intersection -> Manual_Control [order 3] : [park_request == 4]
  Follower_Goto_Intersection -> Leader_Goto_Intersection [order 1] : [park_request ==1]
  Leader_Goto_Intersection -> Enter_ParkingArea [order 2] : [park_request == 3 && ev_x <= 0.2 && ev_x >= -0.2...
      |  && ev_y <=3 && ev_y >= 2 ]
  Follower_Goto_Intersection -> Enter_ParkingArea [order 2] : [park_request == 3 && ev_x <= 0.2 && ev_x >= -0.2...
      |  && ev_y <=3 && ev_y >= 2 ]
  Enter_ParkingArea -> Manual_Control [order 2] : [park_request == 4]
  Enter_ParkingArea -> Find_ParkingSpot [order 1] : [(ev_yaw <=-85 && ev_yaw>= -95)&&...
      | ((parking_spot ==1 && ev_x <=0.30 && ev_x >=-0.30 && ev_y<=1.9 && ev_y >= 1.7) ||...
      |  (parking_spot == 2 && ev_x <= 0.30 && ev_x>= -0.30 && ev_y<=1.6 && ev_y >= 1.45) ||...
      |  (parking_spot ==3 && ev_x <=0.30&& ev_x >= -0.30 && ev_y <=1.2 && ev_y >= 1))]
  Find_ParkingSpot -> Manual_Control [order 2] : [park_request == 4]
  Find_ParkingSpot -> Parking [order 1] : [(parking_spot ==1 && ev_x <= -0.40 && ev_x >= -0.50 && ev_y<=1.7...
      |  && ev_y >= 1.5) || (parking_spot == 2 && ev_x<=-0.70 && ev_x>=-0.80....
      |  && ev_y<=1.3 && ev_y >= 1.1) || (parking_spot ==3 ...
      | && ev_x <=-0.80 && ev_x>= -0.90 && ev_y>=0.70 && ev_y <=0.90)]
  Parking -> Manual_Control [order 2] : [park_request == 4]
  Parking -> Parked [order 1] : [Ultrasonic <= 15]
  Parked -> Manual_Control [order 2] : [park_request == 4]
  Parked -> Reverse_Out_Spot [order 1] : [park_request == 1 || park_request ==2]
  Turn_Car_toInter -> Manual_Control [order 2] : [park_request == 4]
  Goto_Stop_Sign -> Manual_Control [order 2] : [park_request == 4]
  Finished -> Manual_Control [order 2] : [park_request == 4]
  Reverse_Out_Spot -> Manual_Control [order 2] : [park_request == 4]
  Reverse_Out_Spot -> Goto_Stop_Sign [order 1] : [(parking_spot ==1 && ev_x <=0.30 && ev_x >=-0.30 ...
      | && ev_y<=1.9 && ev_y >= 1.4) || (parking_spot == 2 ...
      |   && ev_x <= 0.30 && ev_x>= -0.30 && ev_y<=1.3 ...
      | && ev_y >= 1) || (parking_spot ==3 && ev_x <=0.30...
      | && ev_x >= -0.30 && ev_y <=1 && ev_y >= 0.65)]
  Goto_Stop_Sign -> Turn_Car_toInter [order 1] : [ev_x <= 0.17 && ev_x >= 0.017...
      |  && ev_y >= 0.45 && ev_y <= 0.6]
  Turn_Car_toInter -> Finished [order 1] : [ev_x>=-0.5 && ev_x <= -0.10 && ev_y<=0.36 && ev_y >= 0.3 ]
  data: ev_x input; ev_y input; parking_spot input; Ultrasonic input; linetracking output double; stop output double; reversing output double; turn output double; states output double; park_request input; ev_yaw input; platooning output double; manual_control output double
